simulink model "motor"  (R2020b)
settings: Solver=VariableStepAuto  StartTime=0.0  StopTime=0.25  FixedStep=25E-6  RelTol=1e-3
values from neighbouring files (symbols this model uses):
  B1 = T1/(5890*pi/30)    (= 3.66099603052e-07)    [FullProjectMatlabCode.m]    (also in model.m = km1*I_noload1/w_noload1)
  B2 = T2/(7560*pi/30)    (= 1.3073441754e-07)    [FullProjectMatlabCode.m]    (also in model.m = km2*I_noload2/w_noload2)
  B3 = T3/(18600*pi/30)    (= 1.18657711121e-08)    [FullProjectMatlabCode.m]    (also in model.m = km3*I_noload3/w_noload3)
  DEG = 180/pi    (= 57.2957795131)    [constants.m]
  J1 = 4.98e-7    (= 4.98e-07)    [FullProjectMatlabCode.m]    (also in model.m = INERTIA1)
  J2 = 1.05e-7    (= 1.05e-07)    [FullProjectMatlabCode.m]    (also in model.m = INERTIA2)
  J3 = 0.0162e-7    (= 1.62e-09)    [FullProjectMatlabCode.m]    (also in model.m = INERTIA3)
  kb1 = 1/(SPEED_CONSTANT1/RPM)    [model.m]
  kb2 = 1/(SPEED_CONSTANT2/RPM)    [model.m]
  kb3 = 1/(SPEED_CONSTANT3/RPM)    [model.m]
  kd1 = 0    [model.m]
  kd2 = 0    [model.m]
  kd3 = 0    [model.m]
  ki1 = 0    [model.m]
  ki2 = 0    [model.m]
  ki3 = 0    [model.m]
  km1 = TORQUE_CONSTANT1    [model.m]
  km2 = TORQUE_CONSTANT2    [model.m]
  km3 = TORQUE_CONSTANT3    [model.m]
  kp1 = 0.075*ku1    [model.m]
  kp2 = 0.075*ku2    [model.m]
  kp3 = 0.075*ku3    [model.m]
  La1 = TERMINAL_INDUCTANCE1    [model.m]
  La2 = TERMINAL_INDUCTANCE2    [model.m]
  La3 = TERMINAL_INDUCTANCE3    [model.m]
  Ra1 = TERMINAL_RESISTANCE1    [model.m]
  Ra2 = TERMINAL_RESISTANCE2    [model.m]
  Ra3 = TERMINAL_RESISTANCE3    [model.m]
undefined symbols (not defined in the file or in its folder): A_den1, A_den2, A_den3, A_num1, A_num2, A_num3
libraries: pid_lib x4
settings Model: Creator=lukas  LastModifiedBy=lukas

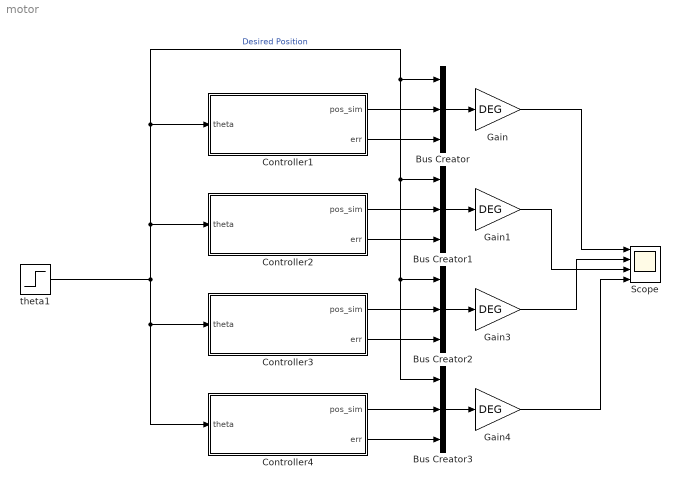
== system motor ==
  Bus Creator{,1..3} (4 alike) : BusCreator  Inputs=3
  Controller1 : Subsystem
  Controller2 : Subsystem
  Controller3 : Subsystem
  Controller4 : Subsystem
  Gain{,1,3..4} (4 alike) : Gain  Gain=DEG
  Scope : Scope  NumInputPorts=4
  theta1 : Step  Time=5e-3  After=1.57  SampleTime=0
  wires:
  Bus Creator/1 -> Gain/1
  Controller1/2(err) -> Bus Creator/3
  Controller1/1(pos_sim) -> Bus Creator/2
  theta1/1 -> Controller4/1(theta), Controller3/1(theta), Controller2/1(theta), Bus Creator3/1, Bus Creator2/1, Bus Creator1/1, Bus Creator/1, Controller1/1(theta)  "Desired Position"
  Controller2/1(pos_sim) -> Bus Creator1/2
  Controller2/2(err) -> Bus Creator1/3
  Bus Creator1/1 -> Gain1/1
  Controller3/1(pos_sim) -> Bus Creator2/2
  Controller3/2(err) -> Bus Creator2/3
  Bus Creator2/1 -> Gain3/1
  Gain/1 -> Scope/1
  Controller4/1(pos_sim) -> Bus Creator3/2
  Bus Creator3/1 -> Gain4/1
  Controller4/2(err) -> Bus Creator3/3
  Gain4/1 -> Scope/4
  Gain1/1 -> Scope/3
  Gain3/1 -> Scope/2

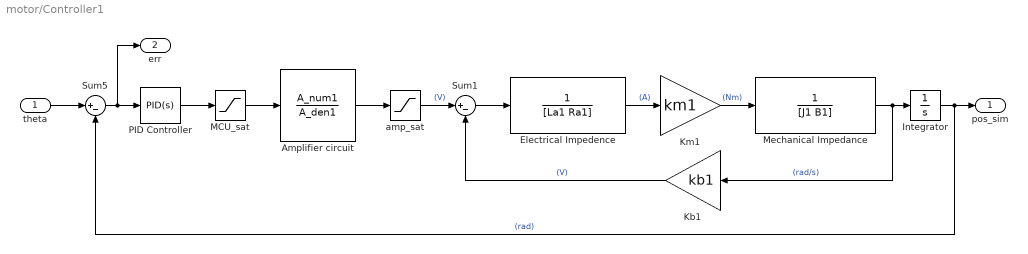
== system motor/Controller1 ==
  theta : Inport
  Amplifier circuit : TransferFcn  Numerator=A_num1  Denominator=A_den1
  Electrical Impedence : TransferFcn  Denominator=[La1 Ra1]
  Integrator : Integrator
  Kb1 : Gain  Gain=kb1
  Km1 : Gain  Gain=km1
  MCU_sat : Saturate  UpperLimit=5  LowerLimit=-5
  Mechanical Impedance : TransferFcn  Denominator=[J1 B1]
  PID Controller : pid_lib/PID Controller  Controller=PID  Form=Parallel  TimeDomain=Continuous-time  UseExternalTs=off  SampleTime=-1  IntegratorMethod=Forward Euler  FilterMethod=Forward Euler  ControllerParametersSource=internal  P=kp1  I=ki1  D=kd1  UseFilter=on  N=100  TunerSelectOption=Transfer Function Based (PID Tuner App)  InitialConditionSource=internal  InitialConditionForIntegrator=0  InitialConditionForFilter=0  DifferentiatorICPrevScaledInput=0  ExternalReset=none  TrackingMode=off  Kt=1  LimitOutput=off  SatLimitsSource=internal  UpperSaturationLimit=inf  LowerSaturationLimit=-inf  LinearizeAsGain=on  AntiWindupMode=none  Kb=1  POutMin=[]  POutMax=[]  IOutMin=[]  IOutMax=[]  DOutMin=[]  DOutMax=[]  NOutMin=[]  NOutMax=[]  SumOutMin=[]  SumOutMax=[]  SaturationOutMin=[]  SaturationOutMax=[]  PParamMin=[]  PParamMax=[]  IParamMin=[]  IParamMax=[]  DParamMin=[]  DParamMax=[]  NParamMin=[]  NParamMax=[]  KbParamMin=[]  KbParamMax=[]  KtParamMin=[]  KtParamMax=[]  KbOutMin=[]  KbOutMax=[]  KtOutMin=[]  KtOutMax=[]  IntegratorOutMin=[]  IntegratorOutMax=[]  FilterOutMin=[]  FilterOutMax=[]  SumI1OutMin=[]  SumI1OutMax=[]  SumI2OutMin=[]  SumI2OutMax=[]  SumI3OutMin=[]  SumI3OutMax=[]  SumI4OutMin=[]  SumI4OutMax=[]  SumDOutMin=[]  SumDOutMax=[]  DifferentiatorOutMin=[]  DifferentiatorOutMax=[]  FilterDiffOutCoefMin=[]  FilterDiffOutCoefMax=[]  ReciprocalOutMin=[]  ReciprocalOutMax=[]  SumDenOutMin=[]  SumDenOutMax=[]  SumNumOutMin=[]  SumNumOutMax=[]  DivideOutMin=[]  DivideOutMax=[]  UdiffTsProdOutMin=[]  UdiffTsProdOutMax=[]  NTsProdOutMin=[]  NTsProdOutMax=[]  UintegralTsProdOutMin=[]  UintegralTsProdOutMax=[]  UngainTsProdOutMin=[]  UngainTsProdOutMax=[]  IntegratorContinuousStateAttributes=''  IntegratorStateMustResolveToSignalObject=off  IntegratorRTWStateStorageClass=Auto  FilterContinuousStateAttributes=''  FilterStateMustResolveToSignalObject=off  FilterRTWStateStorageClass=Auto  ParallelPVariant=InternalParameters  IdealPVariant=Disabled  IVariant=InternalParameters  DVariant=InternalParameters  IntegratorVariant=Continuous  SatVariant=Disabled  AWVariant=Passthrough  PCopyVariant=Disabled  TRVariant=Disabled  FdbkBlocksVariant=Forward  IdealPFdbkVariant=Disabled  SatFdbkVariant=Disabled  DerivativeFilterVariant=ContFilter  NVariant=InternalParameters  NCopyVariant=Disabled  FilterICVariant=InternalICsFilter  IntegratorICVariant=InternalICs  ExternalResetVariant=Disabled  TRSumVariant=Passthrough  SumFdbkVariant=Disabled  SumVariant=Sum_PID  TsampFilterVariant=InternalTs  TsampNgainVariant=Passthrough  TsampIntegralVariant=Passthrough  ExternalSaturationOutDataTypeStr=Inherit: Same as second input
  Sum1 : Sum  Inputs=|+-
  Sum5 : Sum  Inputs=|+-
  amp_sat : Saturate  UpperLimit=12  LowerLimit=-12
  pos_sim : Outport
  err : Outport  Port=2
  wires:
  amp_sat/1 -> Sum1/1  "(V)"
  Electrical Impedence/1 -> Km1/1  "(A)"
  PID Controller/1 -> MCU_sat/1
  Amplifier circuit/1 -> amp_sat/1
  Kb1/1 -> Sum1/2  "(V)"
  Sum1/1 -> Electrical Impedence/1
  MCU_sat/1 -> Amplifier circuit/1
  Km1/1 -> Mechanical Impedance/1  "(Nm)"
  Mechanical Impedance/1 -> Integrator/1, Kb1/1  "(rad/s)"
  Integrator/1 -> pos_sim/1, Sum5/2  "(rad)"
  Sum5/1 -> err/1, PID Controller/1
  theta/1 -> Sum5/1

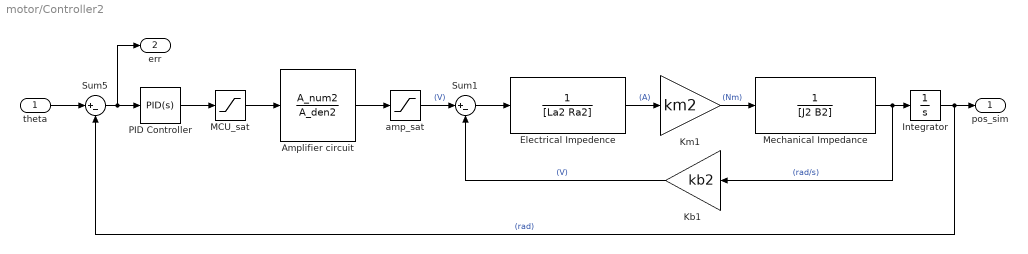
== system motor/Controller2 ==
  theta : Inport
  Amplifier circuit : TransferFcn  Numerator=A_num2  Denominator=A_den2
  Electrical Impedence : TransferFcn  Denominator=[La2 Ra2]
  Integrator : Integrator
  Kb1 : Gain  Gain=kb2
  Km1 : Gain  Gain=km2
  MCU_sat : Saturate  UpperLimit=5  LowerLimit=-5
  Mechanical Impedance : TransferFcn  Denominator=[J2 B2]
  PID Controller : pid_lib/PID Controller  Controller=PID  Form=Parallel  TimeDomain=Continuous-time  UseExternalTs=off  SampleTime=-1  IntegratorMethod=Forward Euler  FilterMethod=Forward Euler  ControllerParametersSource=internal  P=kp2  I=ki2  D=kd2  UseFilter=on  N=100  TunerSelectOption=Transfer Function Based (PID Tuner App)  InitialConditionSource=internal  InitialConditionForIntegrator=0  InitialConditionForFilter=0  DifferentiatorICPrevScaledInput=0  ExternalReset=none  TrackingMode=off  Kt=1  LimitOutput=off  SatLimitsSource=internal  UpperSaturationLimit=inf  LowerSaturationLimit=-inf  LinearizeAsGain=on  AntiWindupMode=none  Kb=1  POutMin=[]  POutMax=[]  IOutMin=[]  IOutMax=[]  DOutMin=[]  DOutMax=[]  NOutMin=[]  NOutMax=[]  SumOutMin=[]  SumOutMax=[]  SaturationOutMin=[]  SaturationOutMax=[]  PParamMin=[]  PParamMax=[]  IParamMin=[]  IParamMax=[]  DParamMin=[]  DParamMax=[]  NParamMin=[]  NParamMax=[]  KbParamMin=[]  KbParamMax=[]  KtParamMin=[]  KtParamMax=[]  KbOutMin=[]  KbOutMax=[]  KtOutMin=[]  KtOutMax=[]  IntegratorOutMin=[]  IntegratorOutMax=[]  FilterOutMin=[]  FilterOutMax=[]  SumI1OutMin=[]  SumI1OutMax=[]  SumI2OutMin=[]  SumI2OutMax=[]  SumI3OutMin=[]  SumI3OutMax=[]  SumI4OutMin=[]  SumI4OutMax=[]  SumDOutMin=[]  SumDOutMax=[]  DifferentiatorOutMin=[]  DifferentiatorOutMax=[]  FilterDiffOutCoefMin=[]  FilterDiffOutCoefMax=[]  ReciprocalOutMin=[]  ReciprocalOutMax=[]  SumDenOutMin=[]  SumDenOutMax=[]  SumNumOutMin=[]  SumNumOutMax=[]  DivideOutMin=[]  DivideOutMax=[]  UdiffTsProdOutMin=[]  UdiffTsProdOutMax=[]  NTsProdOutMin=[]  NTsProdOutMax=[]  UintegralTsProdOutMin=[]  UintegralTsProdOutMax=[]  UngainTsProdOutMin=[]  UngainTsProdOutMax=[]  IntegratorContinuousStateAttributes=''  IntegratorStateMustResolveToSignalObject=off  IntegratorRTWStateStorageClass=Auto  FilterContinuousStateAttributes=''  FilterStateMustResolveToSignalObject=off  FilterRTWStateStorageClass=Auto  ParallelPVariant=InternalParameters  IdealPVariant=Disabled  IVariant=InternalParameters  DVariant=InternalParameters  IntegratorVariant=Continuous  SatVariant=Disabled  AWVariant=Passthrough  PCopyVariant=Disabled  TRVariant=Disabled  FdbkBlocksVariant=Forward  IdealPFdbkVariant=Disabled  SatFdbkVariant=Disabled  DerivativeFilterVariant=ContFilter  NVariant=InternalParameters  NCopyVariant=Disabled  FilterICVariant=InternalICsFilter  IntegratorICVariant=InternalICs  ExternalResetVariant=Disabled  TRSumVariant=Passthrough  SumFdbkVariant=Disabled  SumVariant=Sum_PID  TsampFilterVariant=InternalTs  TsampNgainVariant=Passthrough  TsampIntegralVariant=Passthrough  ExternalSaturationOutDataTypeStr=Inherit: Same as second input
  Sum1 : Sum  Inputs=|+-
  Sum5 : Sum  Inputs=|+-
  amp_sat : Saturate  UpperLimit=12  LowerLimit=-12
  pos_sim : Outport
  err : Outport  Port=2
  wires:
  amp_sat/1 -> Sum1/1  "(V)"
  Electrical Impedence/1 -> Km1/1  "(A)"
  PID Controller/1 -> MCU_sat/1
  Amplifier circuit/1 -> amp_sat/1
  Kb1/1 -> Sum1/2  "(V)"
  Sum1/1 -> Electrical Impedence/1
  MCU_sat/1 -> Amplifier circuit/1
  Km1/1 -> Mechanical Impedance/1  "(Nm)"
  Mechanical Impedance/1 -> Integrator/1, Kb1/1  "(rad/s)"
  Integrator/1 -> pos_sim/1, Sum5/2  "(rad)"
  Sum5/1 -> err/1, PID Controller/1
  theta/1 -> Sum5/1

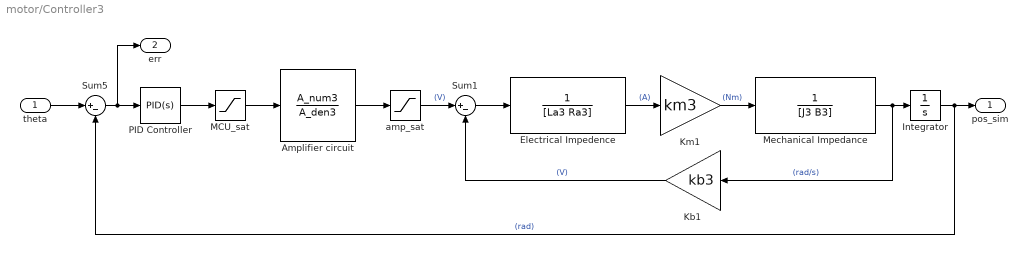
== system motor/Controller3 ==
  theta : Inport
  Amplifier circuit : TransferFcn  Numerator=A_num3  Denominator=A_den3
  Electrical Impedence : TransferFcn  Denominator=[La3 Ra3]
  Integrator : Integrator
  Kb1 : Gain  Gain=kb3
  Km1 : Gain  Gain=km3
  MCU_sat : Saturate  UpperLimit=5  LowerLimit=-5
  Mechanical Impedance : TransferFcn  Denominator=[J3 B3]
  PID Controller : pid_lib/PID Controller  Controller=PID  Form=Parallel  TimeDomain=Continuous-time  UseExternalTs=off  SampleTime=-1  IntegratorMethod=Forward Euler  FilterMethod=Forward Euler  ControllerParametersSource=internal  P=kp3  I=ki3  D=kd3  UseFilter=on  N=100  TunerSelectOption=Transfer Function Based (PID Tuner App)  InitialConditionSource=internal  InitialConditionForIntegrator=0  InitialConditionForFilter=0  DifferentiatorICPrevScaledInput=0  ExternalReset=none  TrackingMode=off  Kt=1  LimitOutput=off  SatLimitsSource=internal  UpperSaturationLimit=inf  LowerSaturationLimit=-inf  LinearizeAsGain=on  AntiWindupMode=none  Kb=1  POutMin=[]  POutMax=[]  IOutMin=[]  IOutMax=[]  DOutMin=[]  DOutMax=[]  NOutMin=[]  NOutMax=[]  SumOutMin=[]  SumOutMax=[]  SaturationOutMin=[]  SaturationOutMax=[]  PParamMin=[]  PParamMax=[]  IParamMin=[]  IParamMax=[]  DParamMin=[]  DParamMax=[]  NParamMin=[]  NParamMax=[]  KbParamMin=[]  KbParamMax=[]  KtParamMin=[]  KtParamMax=[]  KbOutMin=[]  KbOutMax=[]  KtOutMin=[]  KtOutMax=[]  IntegratorOutMin=[]  IntegratorOutMax=[]  FilterOutMin=[]  FilterOutMax=[]  SumI1OutMin=[]  SumI1OutMax=[]  SumI2OutMin=[]  SumI2OutMax=[]  SumI3OutMin=[]  SumI3OutMax=[]  SumI4OutMin=[]  SumI4OutMax=[]  SumDOutMin=[]  SumDOutMax=[]  DifferentiatorOutMin=[]  DifferentiatorOutMax=[]  FilterDiffOutCoefMin=[]  FilterDiffOutCoefMax=[]  ReciprocalOutMin=[]  ReciprocalOutMax=[]  SumDenOutMin=[]  SumDenOutMax=[]  SumNumOutMin=[]  SumNumOutMax=[]  DivideOutMin=[]  DivideOutMax=[]  UdiffTsProdOutMin=[]  UdiffTsProdOutMax=[]  NTsProdOutMin=[]  NTsProdOutMax=[]  UintegralTsProdOutMin=[]  UintegralTsProdOutMax=[]  UngainTsProdOutMin=[]  UngainTsProdOutMax=[]  IntegratorContinuousStateAttributes=''  IntegratorStateMustResolveToSignalObject=off  IntegratorRTWStateStorageClass=Auto  FilterContinuousStateAttributes=''  FilterStateMustResolveToSignalObject=off  FilterRTWStateStorageClass=Auto  ParallelPVariant=InternalParameters  IdealPVariant=Disabled  IVariant=InternalParameters  DVariant=InternalParameters  IntegratorVariant=Continuous  SatVariant=Disabled  AWVariant=Passthrough  PCopyVariant=Disabled  TRVariant=Disabled  FdbkBlocksVariant=Forward  IdealPFdbkVariant=Disabled  SatFdbkVariant=Disabled  DerivativeFilterVariant=ContFilter  NVariant=InternalParameters  NCopyVariant=Disabled  FilterICVariant=InternalICsFilter  IntegratorICVariant=InternalICs  ExternalResetVariant=Disabled  TRSumVariant=Passthrough  SumFdbkVariant=Disabled  SumVariant=Sum_PID  TsampFilterVariant=InternalTs  TsampNgainVariant=Passthrough  TsampIntegralVariant=Passthrough  ExternalSaturationOutDataTypeStr=Inherit: Same as second input
  Sum1 : Sum  Inputs=|+-
  Sum5 : Sum  Inputs=|+-
  amp_sat : Saturate  UpperLimit=6  LowerLimit=-6
  pos_sim : Outport
  err : Outport  Port=2
  wires:
  amp_sat/1 -> Sum1/1  "(V)"
  Electrical Impedence/1 -> Km1/1  "(A)"
  PID Controller/1 -> MCU_sat/1
  Amplifier circuit/1 -> amp_sat/1
  Kb1/1 -> Sum1/2  "(V)"
  Sum1/1 -> Electrical Impedence/1
  MCU_sat/1 -> Amplifier circuit/1
  Km1/1 -> Mechanical Impedance/1  "(Nm)"
  Mechanical Impedance/1 -> Integrator/1, Kb1/1  "(rad/s)"
  Integrator/1 -> pos_sim/1, Sum5/2  "(rad)"
  Sum5/1 -> err/1, PID Controller/1
  theta/1 -> Sum5/1

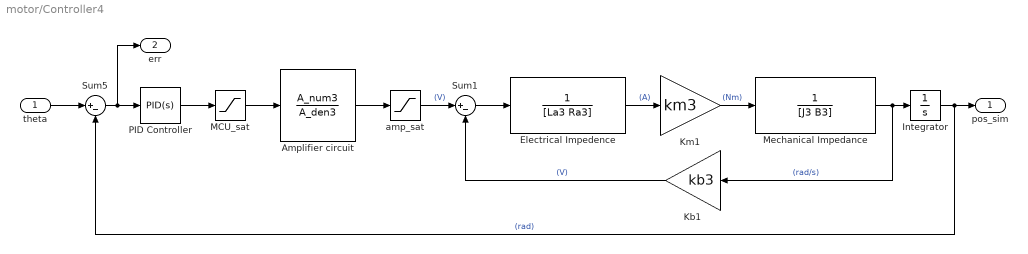
== system motor/Controller4 ==
  theta : Inport
  Amplifier circuit : TransferFcn  Numerator=A_num3  Denominator=A_den3
  Electrical Impedence : TransferFcn  Denominator=[La3 Ra3]
  Integrator : Integrator
  Kb1 : Gain  Gain=kb3
  Km1 : Gain  Gain=km3
  MCU_sat : Saturate  UpperLimit=5  LowerLimit=-5
  Mechanical Impedance : TransferFcn  Denominator=[J3 B3]
  PID Controller : pid_lib/PID Controller  Controller=PID  Form=Parallel  TimeDomain=Continuous-time  UseExternalTs=off  SampleTime=-1  IntegratorMethod=Forward Euler  FilterMethod=Forward Euler  ControllerParametersSource=internal  P=kp3  I=ki3  D=kd3  UseFilter=on  N=100  TunerSelectOption=Transfer Function Based (PID Tuner App)  InitialConditionSource=internal  InitialConditionForIntegrator=0  InitialConditionForFilter=0  DifferentiatorICPrevScaledInput=0  ExternalReset=none  TrackingMode=off  Kt=1  LimitOutput=off  SatLimitsSource=internal  UpperSaturationLimit=inf  LowerSaturationLimit=-inf  LinearizeAsGain=on  AntiWindupMode=none  Kb=1  POutMin=[]  POutMax=[]  IOutMin=[]  IOutMax=[]  DOutMin=[]  DOutMax=[]  NOutMin=[]  NOutMax=[]  SumOutMin=[]  SumOutMax=[]  SaturationOutMin=[]  SaturationOutMax=[]  PParamMin=[]  PParamMax=[]  IParamMin=[]  IParamMax=[]  DParamMin=[]  DParamMax=[]  NParamMin=[]  NParamMax=[]  KbParamMin=[]  KbParamMax=[]  KtParamMin=[]  KtParamMax=[]  KbOutMin=[]  KbOutMax=[]  KtOutMin=[]  KtOutMax=[]  IntegratorOutMin=[]  IntegratorOutMax=[]  FilterOutMin=[]  FilterOutMax=[]  SumI1OutMin=[]  SumI1OutMax=[]  SumI2OutMin=[]  SumI2OutMax=[]  SumI3OutMin=[]  SumI3OutMax=[]  SumI4OutMin=[]  SumI4OutMax=[]  SumDOutMin=[]  SumDOutMax=[]  DifferentiatorOutMin=[]  DifferentiatorOutMax=[]  FilterDiffOutCoefMin=[]  FilterDiffOutCoefMax=[]  ReciprocalOutMin=[]  ReciprocalOutMax=[]  SumDenOutMin=[]  SumDenOutMax=[]  SumNumOutMin=[]  SumNumOutMax=[]  DivideOutMin=[]  DivideOutMax=[]  UdiffTsProdOutMin=[]  UdiffTsProdOutMax=[]  NTsProdOutMin=[]  NTsProdOutMax=[]  UintegralTsProdOutMin=[]  UintegralTsProdOutMax=[]  UngainTsProdOutMin=[]  UngainTsProdOutMax=[]  IntegratorContinuousStateAttributes=''  IntegratorStateMustResolveToSignalObject=off  IntegratorRTWStateStorageClass=Auto  FilterContinuousStateAttributes=''  FilterStateMustResolveToSignalObject=off  FilterRTWStateStorageClass=Auto  ParallelPVariant=InternalParameters  IdealPVariant=Disabled  IVariant=InternalParameters  DVariant=InternalParameters  IntegratorVariant=Continuous  SatVariant=Disabled  AWVariant=Passthrough  PCopyVariant=Disabled  TRVariant=Disabled  FdbkBlocksVariant=Forward  IdealPFdbkVariant=Disabled  SatFdbkVariant=Disabled  DerivativeFilterVariant=ContFilter  NVariant=InternalParameters  NCopyVariant=Disabled  FilterICVariant=InternalICsFilter  IntegratorICVariant=InternalICs  ExternalResetVariant=Disabled  TRSumVariant=Passthrough  SumFdbkVariant=Disabled  SumVariant=Sum_PID  TsampFilterVariant=InternalTs  TsampNgainVariant=Passthrough  TsampIntegralVariant=Passthrough  ExternalSaturationOutDataTypeStr=Inherit: Same as second input
  Sum1 : Sum  Inputs=|+-
  Sum5 : Sum  Inputs=|+-
  amp_sat : Saturate  UpperLimit=6  LowerLimit=-6
  pos_sim : Outport
  err : Outport  Port=2
  wires:
  amp_sat/1 -> Sum1/1  "(V)"
  Electrical Impedence/1 -> Km1/1  "(A)"
  PID Controller/1 -> MCU_sat/1
  Amplifier circuit/1 -> amp_sat/1
  Kb1/1 -> Sum1/2  "(V)"
  Sum1/1 -> Electrical Impedence/1
  MCU_sat/1 -> Amplifier circuit/1
  Km1/1 -> Mechanical Impedance/1  "(Nm)"
  Mechanical Impedance/1 -> Integrator/1, Kb1/1  "(rad/s)"
  Integrator/1 -> pos_sim/1, Sum5/2  "(rad)"
  Sum5/1 -> err/1, PID Controller/1
  theta/1 -> Sum5/1
